simulink model "plant_ElectromagnetUpward_R2016a"  (R2016a)
settings: Solver=ode45  StartTime=0.0  StopTime=10  RelTol=1e-3
undefined symbols (not defined in the file or in its folder): alpha, beta, g, L, m, R, x1bar_init, x2bar_init, x3bar_init
settings Model: Creator=Jon-l  LastModifiedBy=pbarooah
settings DataIOCC: LimitDataPoints=on  SaveFormat=Array  SignalLoggingSaveFormat=ModelDataLogs
settings OptimizationCC: ExpressionDepthLimit=2147483647
settings DebuggingCC: UnderspecifiedInitializationDetection=Classic  MergeDetectMultiDrivingBlocksExec=none  SolverPrmCheckMsg=warning  FcnCallInpInsideContextMsg=EnableAllAsWarning  StateNameClashWarn=warning
settings HardwareCC: ProdBitPerPointer=32  ProdLargestAtomicFloat=None  ProdIntDivRoundTo=Undefined  ProdEndianess=Unspecified  ProdWordSize=32  ProdHWDeviceType=32-bit Generic
settings ModelReferenceCC: PropagateSignalLabelsOutOfModel=off
settings GRTTargetCC: CombineOutputUpdateFcns=off  GRTInterface=on

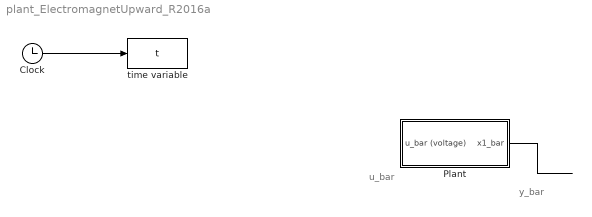
== system plant_ElectromagnetUpward_R2016a ==
  note: u_bar
  note: y_bar
  Clock : Clock
  Plant : Subsystem
  time variable : ToWorkspace  VariableName=t  SaveFormat=Structure  SampleTime=-1
  wires:
  Clock/1 -> time variable/1
  ? -> Plant/1(u_bar (voltage))
  Plant/1(x1_bar) -> ?

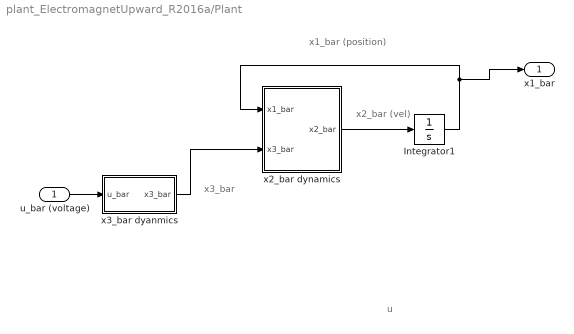
== system plant_ElectromagnetUpward_R2016a/Plant ==
  note: x3_bar
  note: x2_bar
      |  (vel)
  note: u
  note: x1_bar (position)
  u_bar (voltage) : Inport
  Integrator1 : Integrator  InitialCondition=x1bar_init
  x2_bar dynamics : Subsystem
  x3_bar dyanmics : Subsystem
  x1_bar : Outport
  wires:
  Integrator1/1 -> x2_bar dynamics/1(x1_bar), x1_bar/1
  x2_bar dynamics/1(x2_bar) -> Integrator1/1
  x3_bar dyanmics/1(x3_bar) -> x2_bar dynamics/2(x3_bar)
  u_bar (voltage)/1 -> x3_bar dyanmics/1(u_bar)

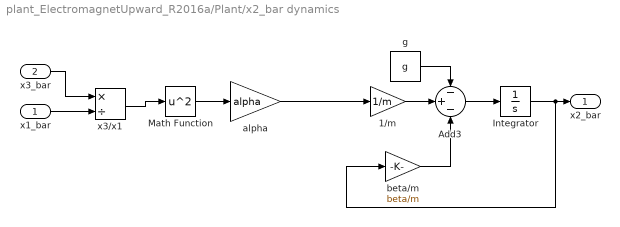
== system plant_ElectromagnetUpward_R2016a/Plant/x2_bar dynamics ==
  x1_bar : Inport
  x3_bar : Inport  Port=2
  1/m : Gain  Gain=1/m
  Add3 : Sum  Inputs=-+-
  Integrator : Integrator  InitialCondition=x2bar_init
  Math Function : Math  Operator=square  SaturateOnIntegerOverflow=on
  alpha : Gain  Gain=alpha
  beta/m : Gain  Gain=beta/m
  g : Constant  Value=g
  x3/x1 : Product  Inputs=*/
  x2_bar : Outport
  wires:
  alpha/1 -> 1/m/1
  1/m/1 -> Add3/2
  Add3/1 -> Integrator/1
  Integrator/1 -> beta/m/1, x2_bar/1
  x1_bar/1 -> x3/x1/2
  x3_bar/1 -> x3/x1/1
  g/1 -> Add3/1
  x3/x1/1 -> Math Function/1
  Math Function/1 -> alpha/1
  beta/m/1 -> Add3/3

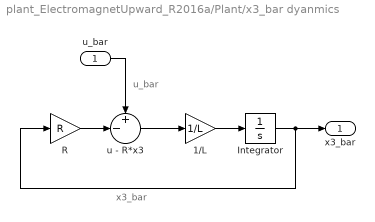
== system plant_ElectromagnetUpward_R2016a/Plant/x3_bar dyanmics ==
  note: u_bar
  note: x3_bar
  u_bar : Inport
  1/L : Gain  Gain=1/L
  Integrator : Integrator  InitialCondition=x3bar_init
  R : Gain  Gain=R
  u - R*x3 : Sum  Inputs=+-|
  x3_bar : Outport
  wires:
  Integrator/1 -> x3_bar/1, R/1
  1/L/1 -> Integrator/1
  u - R*x3/1 -> 1/L/1
  R/1 -> u - R*x3/2
  u_bar/1 -> u - R*x3/1
